simulink model "lab_1_sumlink_module"  (R2023b)
settings: Solver=VariableStepAuto  StartTime=0.0  StopTime=10.0  RelTol=1e-3
settings Model: Creator=ascom  LastModifiedBy=ascom

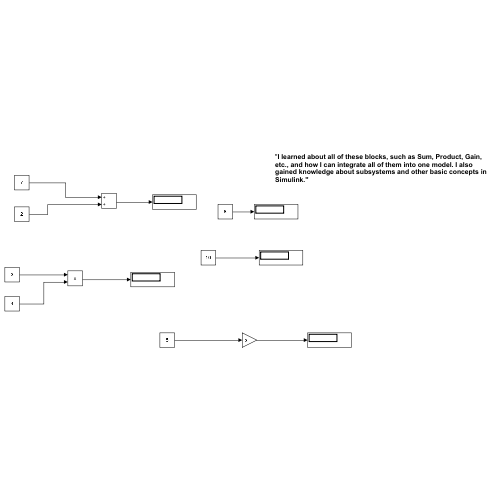
[thumbnail: Simulink's stored preview of the top-level diagram]
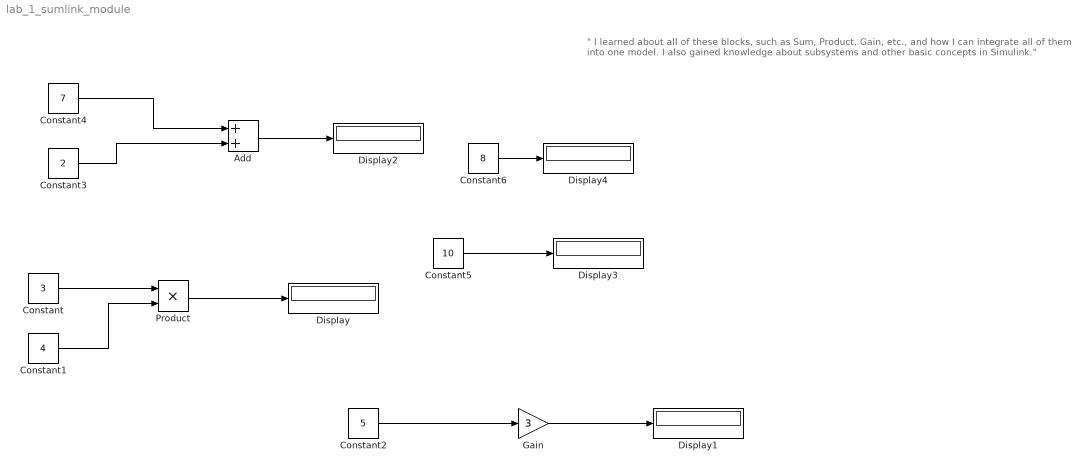
== system lab_1_sumlink_module ==
  note: " I learned about all of these blocks, such as Sum, Product, Gain, etc., and how I can integrate all of them into one model. I also gained knowledge about subsystems and other basic concepts in Simulink."
  Add : Sum
  Constant : Constant  Value=3
  Constant1 : Constant  Value=4
  Constant2 : Constant  Value=5
  Constant3 : Constant  Value=2
  Constant4 : Constant  Value=7
  Constant5 : Constant  Value=10
  Constant6 : Constant  Value=8
  Display{,1..4} (5 alike) : Display
  Gain : Gain  Gain=3
  Product : Product
  wires:
  Constant/1 -> Product/1
  Constant1/1 -> Product/2
  Product/1 -> Display/1
  Constant2/1 -> Gain/1
  Gain/1 -> Display1/1
  Constant4/1 -> Add/1
  Constant3/1 -> Add/2
  Add/1 -> Display2/1
  Constant5/1 -> Display3/1
  Constant6/1 -> Display4/1
